simulink model "kamerazn"  (R2023b)
settings: Solver=VariableStepAuto  StartTime=0.0  StopTime=10  RelTol=1e-8
undefined symbols (not defined in the file): b, g, Gf, l, m, PID, RuS
settings Model: Creator=marija  LastModifiedBy=lvuke
settings SolverCC: AlgebraicLoopSolver=TrustRegion
settings DataIOCC: ReturnWorkspaceOutputs=off
settings DebuggingCC: UnconnectedInputMsg=warning  UnconnectedOutputMsg=warning  UnconnectedLineMsg=warning  ArithmeticOperatorsInVariantConditions=warning
settings ModelReferenceCC: EnableRefExpFcnMdlSchedulingChecks=on
settings SFSimCC: CustomCodeUndefinedFunction=UseInterfaceOnly

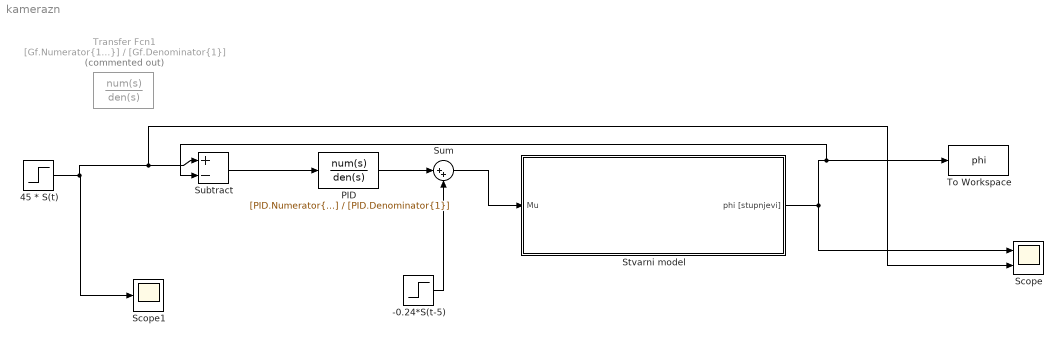
== system kamerazn ==
  -0.24*S(t-5) : Step  Time=5  After=-0.24  SampleTime=0
  45 * S(t) : Step  Time=0  After=45  SampleTime=0
  PID : TransferFcn  Numerator=[PID.Numerator{1}]  Denominator=[PID.Denominator{1}]
  Scope : Scope  NumInputPorts=2
  Scope1 : Scope
  Stvarni model : Subsystem
  Subtract : Sum  Inputs=+-
  Sum : Sum  Inputs=|++
  To Workspace : ToWorkspace  VariableName=phi  SaveFormat=Timeseries  SampleTime=0.001
  Transfer Fcn1 : TransferFcn  Commented=on  Numerator=[Gf.Numerator{1}]  Denominator=[Gf.Denominator{1}]
  wires:
  Stvarni model/1(phi [stupnjevi]) -> Subtract/2, To Workspace/1, Scope/1
  45 * S(t)/1 -> Scope/2, Subtract/1, Scope1/1
  PID/1 -> Sum/1
  Subtract/1 -> PID/1
  -0.24*S(t-5)/1 -> Sum/2
  Sum/1 -> Stvarni model/1(Mu)

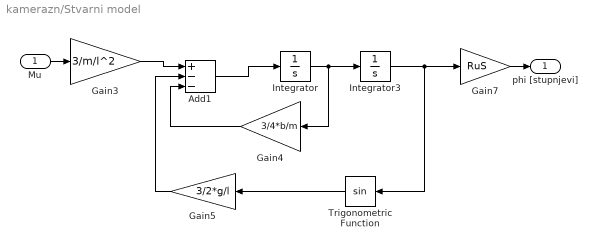
== system kamerazn/Stvarni model ==
  Mu : Inport
  Add1 : Sum  Inputs=+--
  Gain3 : Gain  Gain=3/m/l^2
  Gain4 : Gain  Gain=3/4*b/m
  Gain5 : Gain  Gain=3/2*g/l
  Gain7 : Gain  Gain=RuS
  Integrator : Integrator
  Integrator3 : Integrator
  Trigonometric Function : Trigonometry
  phi [stupnjevi] : Outport  VectorParamsAs1DForOutWhenUnconnected=off
  wires:
  Gain3/1 -> Add1/1
  Gain7/1 -> phi [stupnjevi]/1
  Gain5/1 -> Add1/2
  Gain4/1 -> Add1/3
  Mu/1 -> Gain3/1
  Integrator3/1 -> Trigonometric Function/1, Gain7/1
  Trigonometric Function/1 -> Gain5/1
  Add1/1 -> Integrator/1
  Integrator/1 -> Gain4/1, Integrator3/1
